simulink library "lib_wheel2"  (Simulink 4.1.1)
values from neighbouring files (symbols this model uses):
  logFlag = 1    [advSACompMaskInit.m]    (also in advSACompMaskInitR13.m)
undefined symbols (not defined in the file or in its folder): lib_help, NOTES, veh_air_density, veh_CD, veh_cg_height, veh_FA, veh_front_wt_frac, veh_gravity, veh_roadwheel_radius, veh_rr_a, veh_rr_alpha, veh_rr_b, veh_rr_beta, veh_rr_c, veh_wheelbase, wh_1st_rrc, wh_2nd_rrc, wh_axle_loss_mass, wh_axle_loss_trq, wh_fa_dl_brake_frac, wh_fa_dl_brake_mph, wh_fa_fric_brake_frac, wh_fa_fric_brake_mph, wh_front_active_bool, wh_inertia, wh_max_front_brake_force, wh_max_rear_brake_force, wh_pressure, wh_radius, wh_rear_active_bool, wh_slip, wh_slip_force_coeff
libraries: lib_wheel2 x61, lib_vehicle x2, lib_etc x2, lib_controls x2, lib_wheel x1
(part 9 of 14)

== system lib_wheel2/development/wheel and axle  front/rear <wh> 2 axle --> 1 driveline/wheel & axle model & interface/2 axle --> 1 driveline converter ==
  front req : Inport  Port=1  LatchInput=off
  rear req : Inport  Port=2  LatchInput=off
  ach : Inport  Port=3  LatchInput=off
  Constant : Constant  Value=wh_front_active_bool
  Constant1 : Constant  Value=wh_rear_active_bool
  Constant2 : Constant  Value=wh_front_active_bool
  Constant3 : Constant  Value=wh_rear_active_bool
  Constant4 : Constant  Value=eps
  Constant5 : Constant  Value=0
  Demux : Demux  Outputs=2  BusSelectionMode=off
  Demux1 : Demux  Outputs=2  BusSelectionMode=off
  Demux2 : Demux  Outputs=2  BusSelectionMode=off
  Ground : Ground
  Logical Operator : Logic  Operator=NAND  Inputs=2
  Mux{,1..3} (4 alike) : Mux  Inputs=2
  Product : Product  Inputs=*/  Multiplication=Element-wise(.*)  SaturateOnIntegerOverflow=on
  Product1 : Product  Inputs=2  Multiplication=Element-wise(.*)  SaturateOnIntegerOverflow=on
  Sum : Sum  Inputs=++  SaturateOnIntegerOverflow=on
  Sum1 : Sum  Inputs=+-  SaturateOnIntegerOverflow=on
  Sum2 : Sum  Inputs=++  SaturateOnIntegerOverflow=on
  Switch{,1..6} (7 alike) : Switch  Threshold=eps
  Terminator : Terminator
  req : Outport  Port=1
  front ach : Outport  Port=2
  rear ach : Outport  Port=3
  wires:
  rear req/1 -> Demux1/1, Switch/3
  Constant/1 -> Switch/2, Logical Operator/1
  Switch/1 -> Switch1/1
  Logical Operator/1 -> Switch1/2, Switch2/2, Switch5/2
  Switch1/1 -> req/1
  Mux/1 -> Switch1/3
  Demux1/1 -> Sum/2
  Demux/1 -> Sum/1, Product/1
  Sum/1 -> Mux/1, Sum2/1, Switch6/2
  Demux/2 -> Mux/2
  Demux1/2 -> Terminator/1
  front req/1 -> Demux/1, Switch/1
  Constant1/1 -> Logical Operator/2
  ach/1 -> Demux2/1, Switch2/1, Switch5/1
  Switch3/1 -> front ach/1
  Switch4/1 -> rear ach/1
  Demux2/1 -> Product1/2, Sum1/1
  Product/1 -> Product1/1
  Sum1/1 -> Mux1/1
  Constant3/1 -> Switch4/2
  Constant2/1 -> Switch3/2
  Ground/1 -> Mux3/1
  Mux3/1 -> Switch4/3, Switch3/3
  Mux2/1 -> Switch2/3
  Mux1/1 -> Switch5/3
  Switch2/1 -> Switch3/1
  Switch5/1 -> Switch4/1
  Demux2/2 -> Mux1/2, Mux2/2, Mux3/2
  Constant4/1 -> Sum2/2
  Sum2/1 -> Product/2
  Product1/1 -> Switch6/1
  Switch6/1 -> Mux2/1, Sum1/2
  Constant5/1 -> Switch6/3

== system lib_wheel2/development/wheel and axle  front/rear <wh> 2 axle --> 1 driveline/wheel & axle model & interface/signal annotator ==
  In1 : Inport  Port=1  LatchInput=off
  Demux : Demux  Outputs=2  BusSelectionMode=off
  Mux : Mux  Inputs=2
  Out1 : Outport  Port=1
  wires:
  In1/1 -> Demux/1
  Demux/1 -> Mux/1  "F_traction_r"
  Demux/2 -> Mux/2  "veh_speed_r"
  Mux/1 -> Out1/1

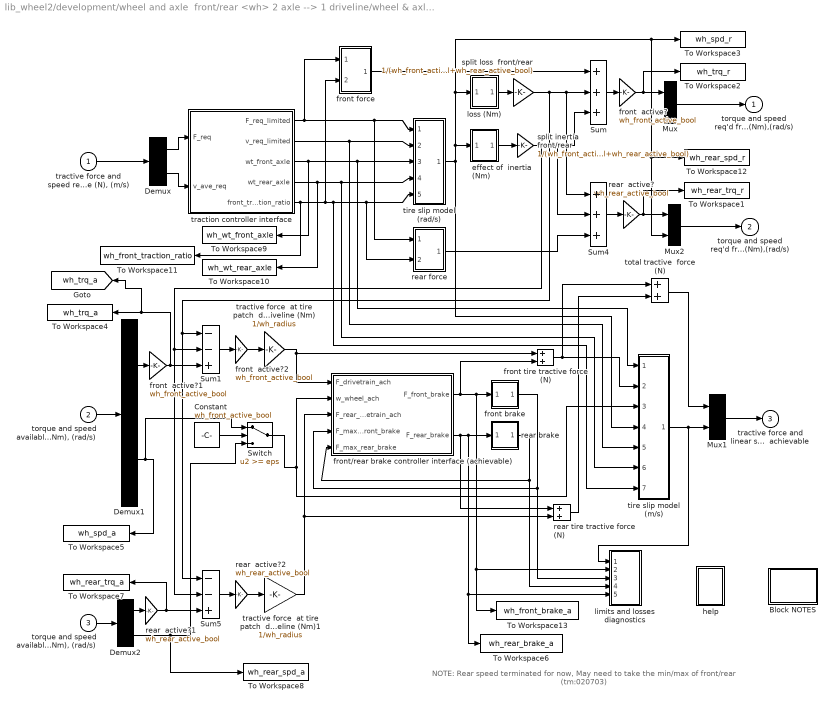
== system lib_wheel2/development/wheel and axle  front/rear <wh> 2 axle --> 1 driveline/wheel & axle model & interface/wheel model ==
  note: NOTE: Rear speed terminated for now, May need to take the min/max of front/rear (tm:020703)
  "tractive force and speed req'd of tire/road interface (N), (m/s)" : Inport  Port=1  LatchInput=off
  "torque and speed available from drivetrain into front axle (Nm), (rad/s)" : Inport  Port=2  LatchInput=off
  "torque and speed available from drivetrain into rear axle (Nm), (rad/s)" : Inport  Port=3  LatchInput=off
  Block NOTES : Subsystem
      settings: RTWFcnNameOpts=Auto  RTWFileNameOpts=Auto
      mask Display: disp('Block\nNOTES')
  Constant : Constant  Value=wh_front_active_bool
  Demux : Demux  Outputs=2  BusSelectionMode=off
  Demux1 : Demux  Outputs=2  BusSelectionMode=off
  Demux2 : Demux  Outputs=2  BusSelectionMode=off
  Mux : Mux  Inputs=2
      settings: DisplayOption=none
  Mux1 : Mux  Inputs=2
      settings: DisplayOption=none
  Mux2 : Mux  Inputs=2
      settings: DisplayOption=none
  Sum : Sum  Inputs=+++  SaturateOnIntegerOverflow=on
  Sum1 : Sum  Inputs=--+  SaturateOnIntegerOverflow=on
  Sum4 : Sum  Inputs=+++  SaturateOnIntegerOverflow=on
  Sum5 : Sum  Inputs=--+  SaturateOnIntegerOverflow=on
  Switch : Switch  Threshold=eps
  To Workspace1 : ToWorkspace  VariableName=wh_rear_trq_r  SampleTime=-1  SaveFormat=Array
  To Workspace10 : ToWorkspace  VariableName=wh_wt_rear_axle  SampleTime=-1  SaveFormat=Array
  To Workspace11 : ToWorkspace  VariableName=wh_front_traction_ratio  SampleTime=-1  SaveFormat=Array
  To Workspace12 : ToWorkspace  VariableName=wh_rear_spd_r  SampleTime=-1  SaveFormat=Array
  To Workspace13 : ToWorkspace  VariableName=wh_front_brake_a  SampleTime=-1  SaveFormat=Array
  To Workspace2 : ToWorkspace  VariableName=wh_trq_r  SampleTime=-1  SaveFormat=Array
  To Workspace3 : ToWorkspace  VariableName=wh_spd_r  SampleTime=-1  SaveFormat=Array
  To Workspace4 : ToWorkspace  VariableName=wh_trq_a  SampleTime=-1  SaveFormat=Array
  To Workspace5 : ToWorkspace  VariableName=wh_spd_a  SampleTime=-1  SaveFormat=Array
  To Workspace6 : ToWorkspace  VariableName=wh_rear_brake_a  SampleTime=-1  SaveFormat=Array
  To Workspace7 : ToWorkspace  VariableName=wh_rear_trq_a  SampleTime=-1  SaveFormat=Array
  To Workspace8 : ToWorkspace  VariableName=wh_rear_spd_a  SampleTime=-1  SaveFormat=Array
  To Workspace9 : ToWorkspace  VariableName=wh_wt_front_axle  SampleTime=-1  SaveFormat=Array
  effect of  inertia (Nm) : Subsystem
      settings: RTWFcnNameOpts=Auto  RTWFileNameOpts=Auto
  front  active? : Gain  Gain=wh_front_active_bool  Multiplication=Element-wise(K.*u)  SaturateOnIntegerOverflow=on
  front  active?1 : Gain  Gain=wh_front_active_bool  Multiplication=Element-wise(K.*u)  SaturateOnIntegerOverflow=on
  front  active?2 : Gain  Gain=wh_front_active_bool  Multiplication=Element-wise(K.*u)  SaturateOnIntegerOverflow=on
  front brake : Subsystem
      settings: RTWFcnNameOpts=Auto  RTWFileNameOpts=Auto
  front force : Subsystem
      settings: RTWFcnNameOpts=Auto  RTWFileNameOpts=Auto
  front tire tractive force (N) : Sum  Inputs=++  SaturateOnIntegerOverflow=on
  front/rear brake controller interface (achievable) : Subsystem
      settings: RTWFcnNameOpts=Auto  RTWFileNameOpts=Auto
  help : Subsystem
      settings: OpenFcn=web(['file:\\\' which('advisor_doc.htm')]);  RTWFcnNameOpts=Auto  RTWFileNameOpts=Auto
      mask Display: image(imread('doc_man.jpg'))
  limits and losses diagnostics : Subsystem
      settings: RTWFcnNameOpts=Auto  RTWFileNameOpts=Auto
  loss (Nm) : Subsystem
      settings: RTWFcnNameOpts=Auto  RTWFileNameOpts=Auto
  rear  active? : Gain  Gain=wh_rear_active_bool  Multiplication=Element-wise(K.*u)  SaturateOnIntegerOverflow=on
  rear  active?1 : Gain  Gain=wh_rear_active_bool  Multiplication=Element-wise(K.*u)  SaturateOnIntegerOverflow=on
  rear  active?2 : Gain  Gain=wh_rear_active_bool  Multiplication=Element-wise(K.*u)  SaturateOnIntegerOverflow=on
  rear brake : Subsystem
      settings: RTWFcnNameOpts=Auto  RTWFileNameOpts=Auto
  rear force : Subsystem
      settings: RTWFcnNameOpts=Auto  RTWFileNameOpts=Auto
  rear tire tractive force (N) : Sum  Inputs=++  SaturateOnIntegerOverflow=on
  split inertia front/rear : Gain  Gain=1/(wh_front_active_bool+wh_rear_active_bool)  Multiplication=Element-wise(K.*u)  SaturateOnIntegerOverflow=on
  split loss  front/rear : Gain  Gain=1/(wh_front_active_bool+wh_rear_active_bool)  Multiplication=Element-wise(K.*u)  SaturateOnIntegerOverflow=on
  tire slip model (m/s) : Subsystem
      settings: RTWFcnNameOpts=Auto  RTWFileNameOpts=Auto
  tire slip model (rad/s) : Subsystem
      settings: RTWFcnNameOpts=Auto  RTWFileNameOpts=Auto
  total tractive  force (N) : Sum  Inputs=++  SaturateOnIntegerOverflow=on
  traction controller interface : Subsystem
      settings: RTWFcnNameOpts=Auto  RTWFileNameOpts=Auto
  tractive force  at tire patch  due to driveline (Nm) : Gain  Gain=1/wh_radius  Multiplication=Element-wise(K.*u)  SaturateOnIntegerOverflow=on
  tractive force  at tire patch  due to driveline (Nm)1 : Gain  Gain=1/wh_radius  Multiplication=Element-wise(K.*u)  SaturateOnIntegerOverflow=on
  torque and speed req'd from drivetrain into front axle (Nm),(rad/s) : Outport  Port=1  InitialOutput=0
  torque and speed req'd from drivetrain into rear axle (Nm),(rad/s) : Outport  Port=2  InitialOutput=0
  tractive force and linear speed  achievable : Outport  Port=3  InitialOutput=0
  tag scope: wh_trq_a=global
  wires:
  traction controller interface/2(v_req_limited) -> tire slip model (rad/s)/2(requested time-step average vehicle speed (m/s)), tire slip model (m/s)/5(vehicle speed required (m/s))
  Demux/2 -> traction controller interface/2(v_ave_req)
  tire slip model (m/s)/1(possible vehicle speed (m/s)) -> Mux1/2, limits and losses diagnostics/1(speed)
  tractive force  at tire patch  due to driveline (Nm)/1 -> front/rear brake controller interface (achievable)/1(F_drivetrain_ach), front tire tractive force (N)/1
  Sum1/1 -> front  active?2/1
  effect of  inertia (Nm)/1(inertia torque (Nm)) -> split inertia front/rear/1
  loss (Nm)/1(drag torque (Nm)) -> split loss  front/rear/1
  "tractive force and speed req'd of tire/road interface (N), (m/s)"/1 -> Demux/1
  tire slip model (rad/s)/1(slip-augmented rotational speed (rad/s)) -> effect of  inertia (Nm)/1(axle input speed (rad/s)), loss (Nm)/1(axle speed (rad/s)), To Workspace3/1, Mux/2, Mux2/2, To Workspace12/1, tire slip model (m/s)/4(axle speed req'd (rad/s))
  front force/1(Out1) -> Sum/1
  Mux1/1 -> tractive force and linear speed  achievable/1
  total tractive  force (N)/1 -> Mux1/1
  "torque and speed available from drivetrain into front axle (Nm), (rad/s)"/1 -> Demux1/1
  front/rear brake controller interface (achievable)/1(F_front_brake) -> front tire tractive force (N)/2, front brake/1(F_brake), limits and losses diagnostics/2(front brake), To Workspace13/1
  front tire tractive force (N)/1 -> tire slip model (m/s)/2(total tractive  force available (N)), total tractive  force (N)/1
  front brake/1(F_brake_max) -> front/rear brake controller interface (achievable)/4(F_max_front_brake), limits and losses diagnostics/3(front brake max)
  rear brake/1(F_brake_max) -> front/rear brake controller interface (achievable)/5(F_max_rear_brake), limits and losses diagnostics/4(rear brake max)
  traction controller interface/3(wt_front_axle) -> tire slip model (rad/s)/3(weight borne by front axle (N)), tire slip model (m/s)/1(weight borne  by front axle (N)), To Workspace9/1
  Mux/1 -> torque and speed req'd from drivetrain into front axle (Nm),(rad/s)/1
  Sum/1 -> front  active?/1
  Demux1/1 -> front  active?1/1
  Switch/1 -> front/rear brake controller interface (achievable)/2(w_wheel_ach), tire slip model (m/s)/3(axle speed available (rad/s))
  traction controller interface/1(F_req_limited) -> rear force/1(In1), tire slip model (rad/s)/1(total tractive  force requested (N)), front force/1(In1)
  front/rear brake controller interface (achievable)/2(F_rear_brake) -> rear tire tractive force (N)/1, rear brake/1(F_brake), limits and losses diagnostics/5(rear brake), To Workspace6/1
  Demux/1 -> traction controller interface/1(F_req)
  traction controller interface/5(front_traction_ratio) -> tire slip model (m/s)/7(front fraction), tire slip model (rad/s)/5(front traction ratio), rear force/2(In2), front force/2(In2), To Workspace11/1
  rear force/1(Out1) -> Sum4/3
  Sum4/1 -> rear  active?/1
  Mux2/1 -> torque and speed req'd from drivetrain into rear axle (Nm),(rad/s)/1
  split loss  front/rear/1 -> Sum/2, Sum4/1, Sum1/1, Sum5/1
  split inertia front/rear/1 -> Sum/3, Sum4/2, Sum1/2, Sum5/2
  traction controller interface/4(wt_rear_axle) -> tire slip model (rad/s)/4(weight borne by  rear axle (N)1), tire slip model (m/s)/6(weight borne by  rear axle (N)), To Workspace10/1
  Sum5/1 -> rear  active?2/1
  "torque and speed available from drivetrain into rear axle (Nm), (rad/s)"/1 -> Demux2/1
  tractive force  at tire patch  due to driveline (Nm)1/1 -> front/rear brake controller interface (achievable)/3(F_rear_drivetrain_ach), rear tire tractive force (N)/2
  rear tire tractive force (N)/1 -> total tractive  force (N)/2
  Demux2/1 -> rear  active?1/1
  Demux2/2 -> To Workspace8/1, Switch/3
  front  active?/1 -> Mux/1, To Workspace2/1
  rear  active?/1 -> To Workspace1/1, Mux2/1
  front  active?1/1 -> To Workspace4/1, [wh_trq_a], Sum1/3
  rear  active?1/1 -> To Workspace7/1, Sum5/3
  rear  active?2/1 -> tractive force  at tire patch  due to driveline (Nm)1/1
  front  active?2/1 -> tractive force  at tire patch  due to driveline (Nm)/1
  Constant/1 -> Switch/2
  Demux1/2 -> Switch/1, To Workspace5/1

== system lib_wheel2/vehicle, wheel, & axle front/rear <wh>/models and interface/slip, braking, traction calcs/config traction control ==
  time-average vehicle speed  req'd (m/s) : Inport  Port=1  LatchInput=off
  vehicle speed at beginning of time  step (m/s) : Inport  Port=2  LatchInput=off
  total tractive force req'd (N) : Inport  Port=3  LatchInput=off
  traction control 2 axle : lib_wheel2/Submodels/traction control 2 axle
      settings: RTWFcnNameOpts=Auto  RTWFileNameOpts=Auto
  req'd force (N) : Outport  Port=1
  req'd speed (m/s) : Outport  Port=2
  weight on front axle (N) : Outport  Port=3
  weight on rear axle (N) : Outport  Port=4
  front/total  traction ratio : Outport  Port=5
  wires:
  time-average vehicle speed  req'd (m/s)/1 -> traction control 2 axle/1
  vehicle speed at beginning of time  step (m/s)/1 -> traction control 2 axle/2
  total tractive force req'd (N)/1 -> traction control 2 axle/3
  traction control 2 axle/1 -> req'd force (N)/1
  traction control 2 axle/2 -> req'd speed (m/s)/1
  traction control 2 axle/3 -> weight on front axle (N)/1
  traction control 2 axle/4 -> weight on rear axle (N)/1
  traction control 2 axle/5 -> front/total  traction ratio/1

== system lib_wheel2/vehicle, wheel, & axle front/rear <wh>/models and interface/vehicle <veh>/Block NOTES ==
  note: Given the tractive force available, this block uses the same equations to determine the achievable speed.
  note: If no drivetrain component ran up against its performance limit during the time step, the achieved speed
      | is taken to be the requested speed.
  note: This block uses the required vehicle speed with vehicle parameters and the previous speed
      | and classic, straightforward equations to determine the tractive force required at the tire/road interface.
  note: A slight simplification, the assumption that (speed_at_end_of_time_step)^2 is roughly equal to
      | (speed_at_end_of_time_step)*(speed_at_beginning_of_time_step), is used to avoid solving
      | a quadratic equation in the solution of v=v(Ftract).
  note: 2003-April-02, Michael O'Keefe
      | Model updated to use a "stand-alone" mask format

== system lib_wheel2/vehicle, wheel, & axle front/rear <wh>/models and interface/vehicle <veh>/enhancedToWorkspace ==
  In1 : Inport  Port=1  LatchInput=off
  To Workspace : ToWorkspace  VariableName=veh_spd_a  SampleTime=-1  SaveFormat=Array
  wires:
  In1/1 -> To Workspace/1

== system lib_wheel2/vehicle, wheel, & axle front/rear <wh>/models and interface/vehicle <veh>/enhancedToWorkspace1 ==
  In1 : Inport  Port=1  LatchInput=off
  To Workspace : ToWorkspace  VariableName=veh_force_a  SampleTime=-1  SaveFormat=Array
  wires:
  In1/1 -> To Workspace/1

== system lib_wheel2/vehicle, wheel, & axle front/rear <wh>/models and interface/vehicle <veh>/enhancedToWorkspace2 ==
  In1 : Inport  Port=1  LatchInput=off
  To Workspace : ToWorkspace  VariableName=veh_spd_r  SampleTime=-1  SaveFormat=Array
  wires:
  In1/1 -> To Workspace/1

== system lib_wheel2/vehicle, wheel, & axle front/rear <wh>/models and interface/vehicle <veh>/enhancedToWorkspace3 ==
  In1 : Inport  Port=1  LatchInput=off
  To Workspace : ToWorkspace  VariableName=veh_force_r  SampleTime=-1  SaveFormat=Array
  wires:
  In1/1 -> To Workspace/1

== system lib_wheel2/vehicle, wheel, & axle front/rear <wh>/models and interface/vehicle <veh>/enhancedToWorkspace4 ==
  In1 : Inport  Port=1  LatchInput=off
  To Workspace : ToWorkspace  VariableName=veh_Fr  SampleTime=-1  SaveFormat=Array
  wires:
  In1/1 -> To Workspace/1

== system lib_wheel2/vehicle, wheel, & axle front/rear <wh>/models and interface/vehicle <veh>/force req'd to accelerate (N) ==
  v(m/s) : Inport  Port=1  LatchInput=off
  v prev : Inport  Port=2  LatchInput=off
  Clock : Clock
      settings: DisplayTime=off  Decimation=10
  Memory : Memory  X0=-0.1  InheritSampleTime=off
      settings: RTWStateStorageClass=Auto
  Product1 : Product  Inputs=**/  Multiplication=Element-wise(.*)  SaturateOnIntegerOverflow=on
  Sum : Sum  Inputs=+-  SaturateOnIntegerOverflow=on
  Sum1 : Sum  Inputs=+-  SaturateOnIntegerOverflow=on
  current veh mass : lib_wheel2/Submodels/current veh mass
      settings: RTWFcnNameOpts=Auto  RTWFileNameOpts=Auto
  (N) : Outport  Port=1  InitialOutput=0
  wires:
  Sum/1 -> Product1/2
  Sum1/1 -> Product1/3
  v(m/s)/1 -> Sum/1
  v prev/1 -> Sum/2
  Product1/1 -> (N)/1
  Memory/1 -> Sum1/2
  Clock/1 -> Memory/1, Sum1/1
  current veh mass/1 -> Product1/1

== system lib_wheel2/vehicle, wheel, & axle front/rear <wh>/models and interface/vehicle <veh>/force req'd to ascend (N) ==
  average vehicle speed over time step (m/s) : Inport  Port=1  LatchInput=off
  Constant : Constant  Value=veh_gravity
  Constant1 : Constant  Value=0
  Product : Product  Inputs=3  Multiplication=Element-wise(.*)  SaturateOnIntegerOverflow=on
  Switch : Switch  Threshold=0
  Trigonometric Function : Trigonometry  Operator=atan  OutputSignalType=auto
  Trigonometric Function1 : Trigonometry  Operator=sin  OutputSignalType=auto
  current veh mass : lib_wheel2/Submodels/current veh mass
      settings: RTWFcnNameOpts=Auto  RTWFileNameOpts=Auto
  (N) : Outport  Port=1  InitialOutput=0
  wires:
  Trigonometric Function/1 -> Trigonometric Function1/1
  Trigonometric Function1/1 -> Product/2
  [grade] -> Trigonometric Function/1
  Constant/1 -> Product/1
  Product/1 -> Switch/1
  Switch/1 -> (N)/1
  Constant1/1 -> Switch/3
  average vehicle speed over time step (m/s)/1 -> Switch/2
  current veh mass/1 -> Product/3

== system lib_wheel2/vehicle, wheel, & axle front/rear <wh>/models and interface/vehicle <veh>/force req'd to overcome aerodynamic drag (N) ==
  average vehicle speed over time step (m/s) : Inport  Port=1  LatchInput=off
  Constant : Constant  Value=veh_air_density*veh_CD*veh_FA*0.5
  Product : Product  Inputs=3  Multiplication=Element-wise(.*)  SaturateOnIntegerOverflow=on
  D aero(N) : Outport  Port=1  InitialOutput=0
  wires:
  average vehicle speed over time step (m/s)/1 -> Product/1, Product/2
  Constant/1 -> Product/3
  Product/1 -> D aero(N)/1

== system lib_wheel2/vehicle, wheel, & axle front/rear <wh>/models and interface/vehicle <veh>/help ==

== system lib_wheel2/vehicle, wheel, & axle front/rear <wh>/models and interface/vehicle <veh>/memory & init speed ==
  note: cyc_mph(1,2)*.447
  note: 2003-April-02, Michael O'Keefe
      |
      | This block passes through the last speed achieved unless this is the initial condition in which
      | case the initial speed value (a supplied control signal) is passed through. For backwards
      | compatibility, the value of v_init should be cyc_mph(1,2)*0.447
  signal in : Inport  Port=1  LatchInput=off
  signal init : Inport  Port=2  LatchInput=off
  Constant : Constant  Value=1
  IC : InitialCondition  Value=0
  Memory : Memory  X0=0  InheritSampleTime=off
      settings: RTWStateStorageClass=Auto
  Switch : Switch  Threshold=0.5
  signal out : Outport  Port=1
  wires:
  signal in/1 -> Memory/1
  Constant/1 -> IC/1
  Memory/1 -> Switch/1
  IC/1 -> Switch/2
  Switch/1 -> signal out/1
  signal init/1 -> Switch/3

== system lib_wheel2/vehicle, wheel, & axle front/rear <wh>/models and interface/vehicle <veh>/record achieved force outputs ==
  note: local tag
  spd_prev : Inport  Port=1  LatchInput=off
  spd : Inport  Port=2  LatchInput=off
  Gain1 : Gain  Gain=0.5  Multiplication=Element-wise(K.*u)  SaturateOnIntegerOverflow=on
  Product{,1..3} (4 alike) : Product  Inputs=2  Multiplication=Element-wise(.*)  SaturateOnIntegerOverflow=on
  Sum2 : Sum  Inputs=++  SaturateOnIntegerOverflow=on
  enhancedToWorkspace : Subsystem  TreatAsAtomicUnit=on  mask(enhancedToWorkspace){generalName=generalName, specificName=pwr_accel_a, logFlag=logFlag}
      mask prompts: generalName "General Name [char-evaluated]"; specificName "Specific Name [char-literal]"; logFlag "Enable flag (1=on,0=off)"
      mask help: A wrapper for the Simulink "To Workspace" block that allows you to evaluate the name of the variable to log to workspace. This is useful to avoid the double logging errors that occur when you pull in two library models that attempt to log to the same variable.
      mask init:
      | enhancedToWsMaker
      settings: CopyFcn=breakLinkCopyFcn  ParentCloseFcn=breakLinkParCloseFcn  RTWFcnNameOpts=Auto  RTWFileNameOpts=Auto
      mask Help:
      | <h2>Enhanced To Workspace Block</h2>
      | <h3>Parameters</h3>
      | <UL>
      | <li><b>General Name:</b> This is the more general name of the variable. Variables are saved to the workspace as <i>generalName_specificName</i>. Note that this is an evaluated variable. If you would like to type in the value directly, it must be surrounded with single quotes. Otherwise you can input the name of a variable containing a char string.</li>
      | <li><b>Specific Name:</b> This is the specific name of the variable. Note that this is input as a char literal (i.e., you don't need quotes).</li>
      | <li><b>Enable Flag:</b> This flag should have the value of 0 or 1. If 0, the variable will not be logged to the workspace. If 1, the variable will be logged. This is done so that variable logging can be turned off to improve speed.</li>
      | </ul>
      | <h3>Overview</h3>
      | <p>The enhanced to workspace block was put together to allow one to dynamically resolve variable names at run time in simulink. This is most powerful when used in conjunction with a masked subsystem to allow multiple instances of that masked subsytem to be used in the same model. The strategy is to set the generalName in the block mask which will allow the block to change the general name for all variable logging on the fly.
      | <h3>Helper Files</h3>
      | <p>Three m-files are required by the enhancedToWorkspace block. These files are located in the &lt; ADVISOR root &gt;/GUI directory :
      | <ul>
      | <li><i>enhancedToWsMaker.m</i> This file runs the mask initialization for the block</li>
      | <li><i>breakLinkCopyFcn.m</i> This file is used by the block callback when the simulink block is copied. It is necessary to break the link to the enhancedToWorkspace similar to the To Workspace block in order for it to be able to configure itself. (Try copying simulink's To Workspace block--it is impossible to make a link)</li>
      | <li><i>breakLinkParCloseFcn.m</i> This file is similar to the breakLinkCopyFcn and is used when a parent system is closed</li>
      | </ul>
      | <hr>
      | 
      | <p>Created 2003-Jan-21, Michael Patrick O'Keefe, NREL</p>
      | 
      | <!--
      | <VARDEF>
      | <H3>var_name</H3>
      | <UL>
      | <LI><B>data type</B> data type here</LI>
      | <LI><B>units</B> units here</LI>
      | <LI><B>vehicle type</B> vehicle type here</LI>
      | <LI><B>description</B> description here</LI>
      | </UL>
      | </VARDEF>
      | -->
      mask Display: disp([generalName,'_',specificName])
  enhancedToWorkspace1 : Subsystem  TreatAsAtomicUnit=on  mask(enhancedToWorkspace){generalName=generalName, specificName=pwr_drag_a, logFlag=logFlag}
      mask prompts: generalName "General Name [char-evaluated]"; specificName "Specific Name [char-literal]"; logFlag "Enable flag (1=on,0=off)"
      mask help: A wrapper for the Simulink "To Workspace" block that allows you to evaluate the name of the variable to log to workspace. This is useful to avoid the double logging errors that occur when you pull in two library models that attempt to log to the same variable.
      mask init:
      | enhancedToWsMaker
      settings: CopyFcn=breakLinkCopyFcn  ParentCloseFcn=breakLinkParCloseFcn  RTWFcnNameOpts=Auto  RTWFileNameOpts=Auto
      mask Help:
      | <h2>Enhanced To Workspace Block</h2>
      | <h3>Parameters</h3>
      | <UL>
      | <li><b>General Name:</b> This is the more general name of the variable. Variables are saved to the workspace as <i>generalName_specificName</i>. Note that this is an evaluated variable. If you would like to type in the value directly, it must be surrounded with single quotes. Otherwise you can input the name of a variable containing a char string.</li>
      | <li><b>Specific Name:</b> This is the specific name of the variable. Note that this is input as a char literal (i.e., you don't need quotes).</li>
      | <li><b>Enable Flag:</b> This flag should have the value of 0 or 1. If 0, the variable will not be logged to the workspace. If 1, the variable will be logged. This is done so that variable logging can be turned off to improve speed.</li>
      | </ul>
      | <h3>Overview</h3>
      | <p>The enhanced to workspace block was put together to allow one to dynamically resolve variable names at run time in simulink. This is most powerful when used in conjunction with a masked subsystem to allow multiple instances of that masked subsytem to be used in the same model. The strategy is to set the generalName in the block mask which will allow the block to change the general name for all variable logging on the fly.
      | <h3>Helper Files</h3>
      | <p>Three m-files are required by the enhancedToWorkspace block. These files are located in the &lt; ADVISOR root &gt;/GUI directory :
      | <ul>
      | <li><i>enhancedToWsMaker.m</i> This file runs the mask initialization for the block</li>
      | <li><i>breakLinkCopyFcn.m</i> This file is used by the block callback when the simulink block is copied. It is necessary to break the link to the enhancedToWorkspace similar to the To Workspace block in order for it to be able to configure itself. (Try copying simulink's To Workspace block--it is impossible to make a link)</li>
      | <li><i>breakLinkParCloseFcn.m</i> This file is similar to the breakLinkCopyFcn and is used when a parent system is closed</li>
      | </ul>
      | <hr>
      | 
      | <p>Created 2003-Jan-21, Michael Patrick O'Keefe, NREL</p>
      | 
      | <!--
      | <VARDEF>
      | <H3>var_name</H3>
      | <UL>
      | <LI><B>data type</B> data type here</LI>
      | <LI><B>units</B> units here</LI>
      | <LI><B>vehicle type</B> vehicle type here</LI>
      | <LI><B>description</B> description here</LI>
      | </UL>
      | </VARDEF>
      | -->
      mask Display: disp([generalName,'_',specificName])
  enhancedToWorkspace2 : Subsystem  TreatAsAtomicUnit=on  mask(enhancedToWorkspace){generalName=generalName, specificName=pwr_ascent_a, logFlag=logFlag}
      mask prompts: generalName "General Name [char-evaluated]"; specificName "Specific Name [char-literal]"; logFlag "Enable flag (1=on,0=off)"
      mask help: A wrapper for the Simulink "To Workspace" block that allows you to evaluate the name of the variable to log to workspace. This is useful to avoid the double logging errors that occur when you pull in two library models that attempt to log to the same variable.
      mask init:
      | enhancedToWsMaker
      settings: CopyFcn=breakLinkCopyFcn  ParentCloseFcn=breakLinkParCloseFcn  RTWFcnNameOpts=Auto  RTWFileNameOpts=Auto
      mask Help:
      | <h2>Enhanced To Workspace Block</h2>
      | <h3>Parameters</h3>
      | <UL>
      | <li><b>General Name:</b> This is the more general name of the variable. Variables are saved to the workspace as <i>generalName_specificName</i>. Note that this is an evaluated variable. If you would like to type in the value directly, it must be surrounded with single quotes. Otherwise you can input the name of a variable containing a char string.</li>
      | <li><b>Specific Name:</b> This is the specific name of the variable. Note that this is input as a char literal (i.e., you don't need quotes).</li>
      | <li><b>Enable Flag:</b> This flag should have the value of 0 or 1. If 0, the variable will not be logged to the workspace. If 1, the variable will be logged. This is done so that variable logging can be turned off to improve speed.</li>
      | </ul>
      | <h3>Overview</h3>
      | <p>The enhanced to workspace block was put together to allow one to dynamically resolve variable names at run time in simulink. This is most powerful when used in conjunction with a masked subsystem to allow multiple instances of that masked subsytem to be used in the same model. The strategy is to set the generalName in the block mask which will allow the block to change the general name for all variable logging on the fly.
      | <h3>Helper Files</h3>
      | <p>Three m-files are required by the enhancedToWorkspace block. These files are located in the &lt; ADVISOR root &gt;/GUI directory :
      | <ul>
      | <li><i>enhancedToWsMaker.m</i> This file runs the mask initialization for the block</li>
      | <li><i>breakLinkCopyFcn.m</i> This file is used by the block callback when the simulink block is copied. It is necessary to break the link to the enhancedToWorkspace similar to the To Workspace block in order for it to be able to configure itself. (Try copying simulink's To Workspace block--it is impossible to make a link)</li>
      | <li><i>breakLinkParCloseFcn.m</i> This file is similar to the breakLinkCopyFcn and is used when a parent system is closed</li>
      | </ul>
      | <hr>
      | 
      | <p>Created 2003-Jan-21, Michael Patrick O'Keefe, NREL</p>
      | 
      | <!--
      | <VARDEF>
      | <H3>var_name</H3>
      | <UL>
      | <LI><B>data type</B> data type here</LI>
      | <LI><B>units</B> units here</LI>
      | <LI><B>vehicle type</B> vehicle type here</LI>
      | <LI><B>description</B> description here</LI>
      | </UL>
      | </VARDEF>
      | -->
      mask Display: disp([generalName,'_',specificName])
  enhancedToWorkspace3 : Subsystem  TreatAsAtomicUnit=on  mask(enhancedToWorkspace){generalName=generalName, specificName=pwr_rr_a, logFlag=logFlag}
      mask prompts: generalName "General Name [char-evaluated]"; specificName "Specific Name [char-literal]"; logFlag "Enable flag (1=on,0=off)"
      mask help: A wrapper for the Simulink "To Workspace" block that allows you to evaluate the name of the variable to log to workspace. This is useful to avoid the double logging errors that occur when you pull in two library models that attempt to log to the same variable.
      mask init:
      | enhancedToWsMaker
      settings: CopyFcn=breakLinkCopyFcn  ParentCloseFcn=breakLinkParCloseFcn  RTWFcnNameOpts=Auto  RTWFileNameOpts=Auto
      mask Help:
      | <h2>Enhanced To Workspace Block</h2>
      | <h3>Parameters</h3>
      | <UL>
      | <li><b>General Name:</b> This is the more general name of the variable. Variables are saved to the workspace as <i>generalName_specificName</i>. Note that this is an evaluated variable. If you would like to type in the value directly, it must be surrounded with single quotes. Otherwise you can input the name of a variable containing a char string.</li>
      | <li><b>Specific Name:</b> This is the specific name of the variable. Note that this is input as a char literal (i.e., you don't need quotes).</li>
      | <li><b>Enable Flag:</b> This flag should have the value of 0 or 1. If 0, the variable will not be logged to the workspace. If 1, the variable will be logged. This is done so that variable logging can be turned off to improve speed.</li>
      | </ul>
      | <h3>Overview</h3>
      | <p>The enhanced to workspace block was put together to allow one to dynamically resolve variable names at run time in simulink. This is most powerful when used in conjunction with a masked subsystem to allow multiple instances of that masked subsytem to be used in the same model. The strategy is to set the generalName in the block mask which will allow the block to change the general name for all variable logging on the fly.
      | <h3>Helper Files</h3>
      | <p>Three m-files are required by the enhancedToWorkspace block. These files are located in the &lt; ADVISOR root &gt;/GUI directory :
      | <ul>
      | <li><i>enhancedToWsMaker.m</i> This file runs the mask initialization for the block</li>
      | <li><i>breakLinkCopyFcn.m</i> This file is used by the block callback when the simulink block is copied. It is necessary to break the link to the enhancedToWorkspace similar to the To Workspace block in order for it to be able to configure itself. (Try copying simulink's To Workspace block--it is impossible to make a link)</li>
      | <li><i>breakLinkParCloseFcn.m</i> This file is similar to the breakLinkCopyFcn and is used when a parent system is closed</li>
      | </ul>
      | <hr>
      | 
      | <p>Created 2003-Jan-21, Michael Patrick O'Keefe, NREL</p>
      | 
      | <!--
      | <VARDEF>
      | <H3>var_name</H3>
      | <UL>
      | <LI><B>data type</B> data type here</LI>
      | <LI><B>units</B> units here</LI>
      | <LI><B>vehicle type</B> vehicle type here</LI>
      | <LI><B>description</B> description here</LI>
      | </UL>
      | </VARDEF>
      | -->
      mask Display: disp([generalName,'_',specificName])
  force req'd to accelerate (N) : lib_wheel2/vehicle, wheel, & axle front//rear <wh>/models and interface/vehicle <veh>/force req'd to accelerate (N)
      settings: RTWFcnNameOpts=Auto  RTWFileNameOpts=Auto
  force req'd to ascend (N) : lib_wheel2/vehicle, wheel, & axle front//rear <wh>/models and interface/vehicle <veh>/force req'd to ascend (N)
      settings: RTWFcnNameOpts=Auto  RTWFileNameOpts=Auto
  force req'd to overcome aerodynamic drag (N) : lib_wheel2/vehicle, wheel, & axle front//rear <wh>/models and interface/vehicle <veh>/force req'd to overcome aerodynamic drag (N)
      settings: RTWFcnNameOpts=Auto  RTWFileNameOpts=Auto
  rolling resistance force : Subsystem  BlockChoice=force req'd to overcome rolling resistance (N)
      settings: AttributesFormatString=%<BlockChoice>  TemplateBlock=lib_wheel2/Submodels/rolling resistance force  MemberBlocks=force req'd to overcome rolling resistance (N),force req'd to overcome rolling resistance (N) j2452  RTWFcnNameOpts=Auto  RTWFileNameOpts=Auto
  tag scope: veh_pwr_accel_a=scoped, veh_pwr_ascent_a=scoped, veh_pwr_drag_a=scoped, veh_pwr_rr_a=scoped
  wires:
  Sum2/1 -> Gain1/1
  spd/1 -> Sum2/1, force req'd to accelerate (N)/1
  spd_prev/1 -> Sum2/2, force req'd to accelerate (N)/2
  force req'd to overcome aerodynamic drag (N)/1 -> Product1/1
  force req'd to ascend (N)/1 -> Product2/1
  rolling resistance force/1(Fr (N)) -> Product3/1
  force req'd to accelerate (N)/1 -> Product/1
  Product/1 -> [veh_pwr_accel_a], enhancedToWorkspace/1(In1)
  Product1/1 -> [veh_pwr_drag_a], enhancedToWorkspace1/1(In1)
  [vel_ave] -> Product/2
  [vel_ave] -> Product1/2
  [vel_ave] -> Product2/2
  Product2/1 -> [veh_pwr_ascent_a], enhancedToWorkspace2/1(In1)
  [vel_ave] -> Product3/2
  Product3/1 -> [veh_pwr_rr_a], enhancedToWorkspace3/1(In1)
  Gain1/1 -> force req'd to ascend (N)/1, rolling resistance force/1(average vehicle speed over time step (m/s)), [vel_ave], force req'd to overcome aerodynamic drag (N)/1

== system lib_wheel2/vehicle, wheel, & axle front/rear <wh>/models and interface/vehicle <veh>/rolling resistance force ==
  average vehicle speed over time step (m/s) : Inport  Port=1  LatchInput=off
  force req'd to overcome rolling resistance (N) : lib_wheel2/Submodels/force req'd to overcome rolling resistance (N)
      settings: RTWFcnNameOpts=Auto  RTWFileNameOpts=Auto
  Fr (N) : Outport  Port=1
  wires:
  average vehicle speed over time step (m/s)/1 -> force req'd to overcome rolling resistance (N)/1
  force req'd to overcome rolling resistance (N)/1 -> Fr (N)/1

== system lib_wheel2/vehicle, wheel, & axle front/rear <wh>/models and interface/vehicle <veh>/vehicle speed ==
  vehicle speed at beginning of time step (m/s) : Inport  Port=1  LatchInput=off
  "available tractive force and linear speed (N), (m/s)" : Inport  Port=2  LatchInput=off
  vehicle speed (m/s) : lib_wheel2/Submodels/vehicle speed (m//s)
      settings: RTWFcnNameOpts=Auto  RTWFileNameOpts=Auto
  vehicle speed achievable at end of time step (m/s) : Outport  Port=1
  wires:
  vehicle speed at beginning of time step (m/s)/1 -> vehicle speed (m/s)/1
  "available tractive force and linear speed (N), (m/s)"/1 -> vehicle speed (m/s)/2
  vehicle speed (m/s)/1 -> vehicle speed achievable at end of time step (m/s)/1

== system lib_wheel2/vehicle, wheel, & axle front/rear <wh>/models and interface/wheel and axle  front/rear <wh>/Block NOTES ==
  note: This block determines the required axle torque and speed given the tractive force and
      | speed required to meet the trace in the top blocks, and determines the available tractive
      | force and possible vehicle speed given the drivetrain-input torque and rotational speed
      | in the bottom blocks.  The "wheel control" blocks apply the braking strategy and ensure
      | that accelerations beyond the capability of the tires are not requested.

== system lib_wheel2/vehicle, wheel, & axle front/rear <wh>/models and interface/wheel and axle  front/rear <wh>/effect of  inertia (Nm) ==
  note: This block computes the torque required to overcome the inertia of the
      | wheels and axle.
  axle input speed (rad/s) : Inport  Port=1  LatchInput=off
  Constant : Constant  Value=wh_inertia
  Product : Product  Inputs=2  Multiplication=Element-wise(.*)  SaturateOnIntegerOverflow=on
  d/dt : Derivative
  inertia torque (Nm) : Outport  Port=1  InitialOutput=0
  wires:
  d/dt/1 -> Product/1
  axle input speed (rad/s)/1 -> d/dt/1
  Constant/1 -> Product/2
  Product/1 -> inertia torque (Nm)/1

== system lib_wheel2/vehicle, wheel, & axle front/rear <wh>/models and interface/wheel and axle  front/rear <wh>/enhancedToWorkspace ==
  In1 : Inport  Port=1  LatchInput=off
  To Workspace : ToWorkspace  VariableName=wh_rear_spd_a  SampleTime=-1  SaveFormat=Array
  wires:
  In1/1 -> To Workspace/1

== system lib_wheel2/vehicle, wheel, & axle front/rear <wh>/models and interface/wheel and axle  front/rear <wh>/enhancedToWorkspace1 ==
  In1 : Inport  Port=1  LatchInput=off
  To Workspace : ToWorkspace  VariableName=wh_wt_front_axle  SampleTime=-1  SaveFormat=Array
  wires:
  In1/1 -> To Workspace/1

== system lib_wheel2/vehicle, wheel, & axle front/rear <wh>/models and interface/wheel and axle  front/rear <wh>/enhancedToWorkspace10 ==
  In1 : Inport  Port=1  LatchInput=off
  To Workspace : ToWorkspace  VariableName=wh_trq_r  SampleTime=-1  SaveFormat=Array
  wires:
  In1/1 -> To Workspace/1

== system lib_wheel2/vehicle, wheel, & axle front/rear <wh>/models and interface/wheel and axle  front/rear <wh>/enhancedToWorkspace11 ==
  In1 : Inport  Port=1  LatchInput=off
  To Workspace : ToWorkspace  VariableName=wh_rear_brake_a  SampleTime=-1  SaveFormat=Array
  wires:
  In1/1 -> To Workspace/1

== system lib_wheel2/vehicle, wheel, & axle front/rear <wh>/models and interface/wheel and axle  front/rear <wh>/enhancedToWorkspace12 ==
  In1 : Inport  Port=1  LatchInput=off
  To Workspace : ToWorkspace  VariableName=wh_front_brake_a  SampleTime=-1  SaveFormat=Array
  wires:
  In1/1 -> To Workspace/1

== system lib_wheel2/vehicle, wheel, & axle front/rear <wh>/models and interface/wheel and axle  front/rear <wh>/enhancedToWorkspace2 ==
  In1 : Inport  Port=1  LatchInput=off
  To Workspace : ToWorkspace  VariableName=wh_front_traction_ratio  SampleTime=-1  SaveFormat=Array
  wires:
  In1/1 -> To Workspace/1

== system lib_wheel2/vehicle, wheel, & axle front/rear <wh>/models and interface/wheel and axle  front/rear <wh>/enhancedToWorkspace3 ==
  In1 : Inport  Port=1  LatchInput=off
  To Workspace : ToWorkspace  VariableName=wh_wt_rear_axle  SampleTime=-1  SaveFormat=Array
  wires:
  In1/1 -> To Workspace/1

== system lib_wheel2/vehicle, wheel, & axle front/rear <wh>/models and interface/wheel and axle  front/rear <wh>/enhancedToWorkspace4 ==
  In1 : Inport  Port=1  LatchInput=off
  To Workspace : ToWorkspace  VariableName=wh_trq_a  SampleTime=-1  SaveFormat=Array
  wires:
  In1/1 -> To Workspace/1

== system lib_wheel2/vehicle, wheel, & axle front/rear <wh>/models and interface/wheel and axle  front/rear <wh>/enhancedToWorkspace5 ==
  In1 : Inport  Port=1  LatchInput=off
  To Workspace : ToWorkspace  VariableName=wh_spd_a  SampleTime=-1  SaveFormat=Array
  wires:
  In1/1 -> To Workspace/1

== system lib_wheel2/vehicle, wheel, & axle front/rear <wh>/models and interface/wheel and axle  front/rear <wh>/enhancedToWorkspace6 ==
  In1 : Inport  Port=1  LatchInput=off
  To Workspace : ToWorkspace  VariableName=wh_rear_trq_a  SampleTime=-1  SaveFormat=Array
  wires:
  In1/1 -> To Workspace/1

== system lib_wheel2/vehicle, wheel, & axle front/rear <wh>/models and interface/wheel and axle  front/rear <wh>/enhancedToWorkspace7 ==
  In1 : Inport  Port=1  LatchInput=off
  To Workspace : ToWorkspace  VariableName=wh_rear_spd_r  SampleTime=-1  SaveFormat=Array
  wires:
  In1/1 -> To Workspace/1

== system lib_wheel2/vehicle, wheel, & axle front/rear <wh>/models and interface/wheel and axle  front/rear <wh>/enhancedToWorkspace8 ==
  In1 : Inport  Port=1  LatchInput=off
  To Workspace : ToWorkspace  VariableName=wh_rear_trq_r  SampleTime=-1  SaveFormat=Array
  wires:
  In1/1 -> To Workspace/1

== system lib_wheel2/vehicle, wheel, & axle front/rear <wh>/models and interface/wheel and axle  front/rear <wh>/enhancedToWorkspace9 ==
  In1 : Inport  Port=1  LatchInput=off
  To Workspace : ToWorkspace  VariableName=wh_spd_r  SampleTime=-1  SaveFormat=Array
  wires:
  In1/1 -> To Workspace/1

== system lib_wheel2/vehicle, wheel, & axle front/rear <wh>/models and interface/wheel and axle  front/rear <wh>/front brake ==
  F_brake : Inport  Port=1  LatchInput=off
  Constant : Constant  Value=wh_max_front_brake_force
  Terminator : Terminator
  F_brake_max : Outport  Port=1  InitialOutput=0
  wires:
  F_brake/1 -> Terminator/1
  Constant/1 -> F_brake_max/1

== system lib_wheel2/vehicle, wheel, & axle front/rear <wh>/models and interface/wheel and axle  front/rear <wh>/front force ==
  In1 : Inport  Orientation=up  Port=1  LatchInput=off
  In2 : Inport  Port=2  LatchInput=off
  Product1 : Product  Inputs=2  Multiplication=Element-wise(.*)  SaturateOnIntegerOverflow=on
  Sum2 : Sum  Inputs=-+  SaturateOnIntegerOverflow=on
  brake request  controller interface : Subsystem
      settings: RTWFcnNameOpts=Auto  RTWFileNameOpts=Auto
  enhancedToWorkspace11 : Subsystem  TreatAsAtomicUnit=on  mask(enhancedToWorkspace){generalName=generalName01, specificName=front_brake_r, logFlag=logFlag}
      mask prompts: generalName "General Name [char-evaluated]"; specificName "Specific Name [char-literal]"; logFlag "Enable flag (1=on,0=off)"
      mask help: A wrapper for the Simulink "To Workspace" block that allows you to evaluate the name of the variable to log to workspace. This is useful to avoid the double logging errors that occur when you pull in two library models that attempt to log to the same variable.
      mask init:
      | enhancedToWsMaker
      settings: CopyFcn=breakLinkCopyFcn  ParentCloseFcn=breakLinkParCloseFcn  RTWFcnNameOpts=Auto  RTWFileNameOpts=Auto
      mask Help:
      | <h2>Enhanced To Workspace Block</h2>
      | <h3>Parameters</h3>
      | <UL>
      | <li><b>General Name:</b> This is the more general name of the variable. Variables are saved to the workspace as <i>generalName_specificName</i>. Note that this is an evaluated variable. If you would like to type in the value directly, it must be surrounded with single quotes. Otherwise you can input the name of a variable containing a char string.</li>
      | <li><b>Specific Name:</b> This is the specific name of the variable. Note that this is input as a char literal (i.e., you don't need quotes).</li>
      | <li><b>Enable Flag:</b> This flag should have the value of 0 or 1. If 0, the variable will not be logged to the workspace. If 1, the variable will be logged. This is done so that variable logging can be turned off to improve speed.</li>
      | </ul>
      | <h3>Overview</h3>
      | <p>The enhanced to workspace block was put together to allow one to dynamically resolve variable names at run time in simulink. This is most powerful when used in conjunction with a masked subsystem to allow multiple instances of that masked subsytem to be used in the same model. The strategy is to set the generalName in the block mask which will allow the block to change the general name for all variable logging on the fly.
      | <h3>Helper Files</h3>
      | <p>Three m-files are required by the enhancedToWorkspace block. These files are located in the &lt; ADVISOR root &gt;/GUI directory :
      | <ul>
      | <li><i>enhancedToWsMaker.m</i> This file runs the mask initialization for the block</li>
      | <li><i>breakLinkCopyFcn.m</i> This file is used by the block callback when the simulink block is copied. It is necessary to break the link to the enhancedToWorkspace similar to the To Workspace block in order for it to be able to configure itself. (Try copying simulink's To Workspace block--it is impossible to make a link)</li>
      | <li><i>breakLinkParCloseFcn.m</i> This file is similar to the breakLinkCopyFcn and is used when a parent system is closed</li>
      | </ul>
      | <hr>
      | 
      | <p>Created 2003-Jan-21, Michael Patrick O'Keefe, NREL</p>
      | 
      | <!--
      | <VARDEF>
      | <H3>var_name</H3>
      | <UL>
      | <LI><B>data type</B> data type here</LI>
      | <LI><B>units</B> units here</LI>
      | <LI><B>vehicle type</B> vehicle type here</LI>
      | <LI><B>description</B> description here</LI>
      | </UL>
      | </VARDEF>
      | -->
      mask Display: disp([generalName,'_',specificName])
  tractive torque req/d of drivetrain (Nm) : Gain  Gain=wh_radius  Multiplication=Element-wise(K.*u)  SaturateOnIntegerOverflow=on
  Out1 : Outport  Port=1
  wires:
  brake request  controller interface/1(F_front_brake_req) -> Sum2/1, enhancedToWorkspace11/1(In1)
  Sum2/1 -> tractive torque req/d of drivetrain (Nm)/1
  Product1/1 -> Sum2/2
  In1/1 -> Product1/1
  In2/1 -> Product1/2
  tractive torque req/d of drivetrain (Nm)/1 -> Out1/1

== system lib_wheel2/vehicle, wheel, & axle front/rear <wh>/models and interface/wheel and axle  front/rear <wh>/front/rear brake controller interface (achievable) ==
  F_drivetrain_ach : Inport  Port=1  LatchInput=off
  w_wheel_ach : Inport  Port=2  LatchInput=off
  F_rear_drivetrain_ach : Inport  Port=3  LatchInput=off
  F_max_front_brake : Inport  Port=4  LatchInput=off
  F_max_rear_brake : Inport  Port=5  LatchInput=off
  F_front_brake : Outport  Port=1  InitialOutput=0
  F_rear_brake : Outport  Port=2  InitialOutput=0
  tag scope: F_drivetrain_ach=scoped, F_max_front_brake=scoped, F_max_rear_brake=scoped, F_rear_drivetrain_ach=scoped, w_wheel_ach=scoped
  wires:
  [F_rear_brake] -> F_rear_brake/1
  [F_front_brake] -> F_front_brake/1
  w_wheel_ach/1 -> [w_wheel_ach]
  F_drivetrain_ach/1 -> [F_drivetrain_ach]
  F_max_front_brake/1 -> [F_max_front_brake]
  F_max_rear_brake/1 -> [F_max_rear_brake]
  F_rear_drivetrain_ach/1 -> [F_rear_drivetrain_ach]

== system lib_wheel2/vehicle, wheel, & axle front/rear <wh>/models and interface/wheel and axle  front/rear <wh>/help ==
